simulink model "ex3_scrambler_interleaver_ber"  (R2017a)
settings: Solver=FixedStepAuto  StartTime=0  StopTime=100e-3  RelTol=1e-3
model workspace (MAT data in the model file):
  M = 4
  Rb = 1000
  beta = 0.3
  osf = 16
  span = 12
libraries: commsequence2 x2, commblkintrlv2 x2, commsink2 x1, commrandsrc3 x1
settings Model: Creator=root  LastModifiedBy=root

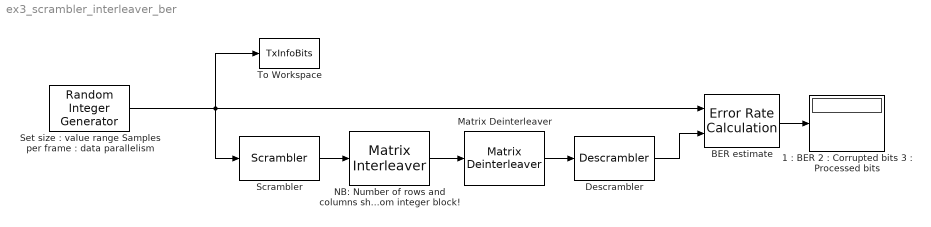
== system ex3_scrambler_interleaver_ber ==
  "1 : BER 2 : Corrupted bits 3 : Processed bits" : Display
  BER estimate : commsink2/Error Rate Calculation  N=0  st_delay=0  cp_mode=Entire frame  subframe=[]  PMode=Port  WsName=ErrorVec  RsMode2=off  stop=off  numErr=100  maxBits=1e6
  Descrambler : commsequence2/Descrambler  M=4  poly='1 + z^-1 + z^-2 + z^-4'  iniStaSource=Dialog Parameter  ini_sta=[0 1 2 3]  resetViaPort=off
      settings: SourceProductName=Communications System Toolbox  SourceProductBaseCode=CM
  Matrix Deinterleaver : commblkintrlv2/Matrix Deinterleaver  Nrows=2  Ncols=4
      settings: SourceProductName=Communications System Toolbox  SourceProductBaseCode=CM
  NB: Number of rows and columns shall match the sampleper-frame in the random integer block! : commblkintrlv2/Matrix Interleaver  Nrows=2  Ncols=4
      settings: SourceProductName=Communications System Toolbox  SourceProductBaseCode=CM
  Scrambler : commsequence2/Scrambler  M=4  poly='1 + z^-1 + z^-2 + z^-4'  iniStaSource=Dialog Parameter  ini_sta=[0 1 2 3]  resetViaPort=off
      settings: SourceProductName=Communications System Toolbox  SourceProductBaseCode=CM
  "Set size : value range Samples per frame : data parallelism" : commrandsrc3/Random Integer Generator  SetSize=2  SeedSource=Auto  Seed=1922  SampleTime=1/Rb  SamplesPerFrame=8  OutputDataType=uint8  SimulateUsing=Interpreted execution
  To Workspace : ToWorkspace  VariableName=TxInfoBits  SaveFormat=Timeseries  SampleTime=-1
  wires:
  "Set size : value range Samples per frame : data parallelism"/1 -> To Workspace/1, BER estimate/1, Scrambler/1
  BER estimate/1 -> "1 : BER 2 : Corrupted bits 3 : Processed bits"/1
  Descrambler/1 -> BER estimate/2
  Scrambler/1 -> NB: Number of rows and columns shall match the sampleper-frame in the random integer block!/1
  NB: Number of rows and columns shall match the sampleper-frame in the random integer block!/1 -> Matrix Deinterleaver/1
  Matrix Deinterleaver/1 -> Descrambler/1
